simulink model "arduino_I2C_hmc5983"  (R2019b)
settings: Solver=FixedStepAuto  StartTime=0.0  StopTime=120  RelTol=1e-3  EnableMultiTasking=on
model workspace (MAT data in the model file):
  craVal = 144
  crbVal = 224
  modeVal = 0
  slaveaddress = 30
libraries: arduinolib x18, simulink x1
settings Model: SILPILModeSetting=veronly  ExtModeTrigDuration=2  OrderedModelArguments=off  Creator=Hirotoshi Maeda  LastModifiedBy=Hirotoshi Maeda
settings OptimizationCC: EnhancedBackFolding=on  PassReuseOutputArgsAs=Individual arguments  ZeroExternalMemoryAtStartup=off  ZeroInternalMemoryAtStartup=off  MaxStackSize=64  OptimizeBlockOrder=speed  DifferentSizesBufferReuse=on  OptimizationCustomize=off  EfficientTunableParamExpr=on
settings DebuggingCC: ParameterTunabilityLossMsg=error
settings HardwareCC: ProdBitPerInt=16  ProdBitPerPointer=16  ProdBitPerSizeT=16  ProdBitPerPtrDiffT=16  ProdLargestAtomicFloat=None  ProdWordSize=8  ProdHWDeviceType=Atmel->AVR  UseSimulinkCoderFeatures=off
settings SFSimCC: MATLABDynamicMemAlloc=off
settings RTWCC: SystemTargetFile=ert.tlc  HardwareBoard=Arduino Uno  TLCOptions=-aInlineSetEventsForThisBaseRateFcn=TLC_FALSE -aSuppressMultiTaskScheduler=TLC_FALSE -aRateBasedStepFcn=1  TemplateMakefile=ert_default_tmf  RTWVerbose=off  Toolchain=Arduino AVR  BuildConfiguration=Faster Runs  IncludeHyperlinkInReport=on
settings CodeAppCC: ForceParamTrailComments=on  OperatorAnnotations=on  SimulinkDataObjDesc=on  SFDataObjDesc=on  MangleLength=10  InsertBlockDesc=on
settings ERTTargetCC: SupportContinuousTime=on  SupportVariableSizeSignals=on  ExtMode=on  ExtModeStaticAllocSize=250  ExtModeMexArgs='127.0.0.1' 0 17725  ERTSrcFileBannerTemplate=codertarget_code_template.cgt  ERTHdrFileBannerTemplate=codertarget_code_template.cgt  ERTDataSrcFileTemplate=codertarget_code_template.cgt  ERTDataHdrFileTemplate=codertarget_code_template.cgt

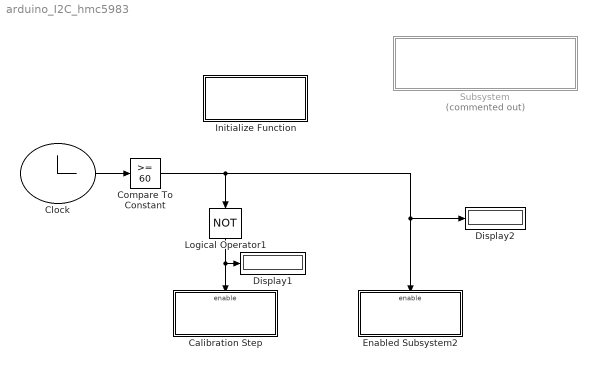
== system arduino_I2C_hmc5983 ==
  "Calibration Step " : Subsystem  Priority=3  TreatAsAtomicUnit=on
  Clock : Clock
  Compare To Constant : simulink/Logic and Bit Operations/Compare To Constant  relop=>=  const=60  OutDataTypeStr=boolean
  Display1 : Display
  Display2 : Display
  Enabled Subsystem2 : Subsystem  Priority=3  TreatAsAtomicUnit=on
  Initialize Function : Subsystem  TreatAsAtomicUnit=on
  Logical Operator1 : Logic  Operator=NOT  AllPortsSameDT=off  OutDataTypeStr=boolean
  Subsystem : Subsystem  Commented=on
  wires:
  Compare To Constant/1 -> Logical Operator1/1, Enabled Subsystem2/Enable, Display2/1
  Clock/1 -> Compare To Constant/1
  Logical Operator1/1 -> "Calibration Step "/Enable, Display1/1

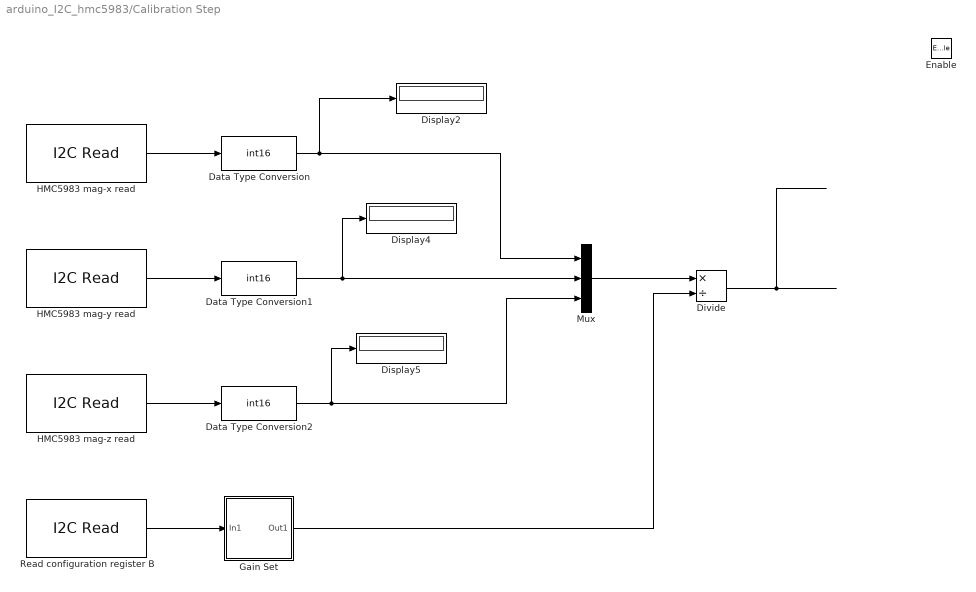
== system arduino_I2C_hmc5983/Calibration Step  ==
  Enable : EnablePort
  Data Type Conversion : DataTypeConversion  OutDataTypeStr=int16
  Data Type Conversion1 : DataTypeConversion  OutDataTypeStr=int16
  Data Type Conversion2 : DataTypeConversion  OutDataTypeStr=int16
  Display2 : Display
      settings: Format=hex (Stored Integer)
  Display4 : Display
      settings: Format=hex (Stored Integer)
  Display5 : Display
      settings: Format=hex (Stored Integer)
  Divide : Product  Inputs=*/
  Gain Set : Subsystem
  HMC5983 mag-x read : arduinolib/I2C Read  I2CModule=0  Mode=Master  SlaveAddress=slaveaddress  SlaveByteOrder=BigEndian  Direction=Receiver  RegisterAddressMode=on  RegisterAddress=hex2dec('03')  SlaveDataType=int16  DataLength=1  NoAck=off  RepeatedStart=off  OutputStatus=off  blockPlatform=ARDUINO  SampleTime=.1
      settings: SourceProductName=Simulink Support Package for Arduino Hardware  SourceProductBaseCode=ARDUINO
  HMC5983 mag-y read : arduinolib/I2C Read  I2CModule=0  Mode=Master  SlaveAddress=slaveaddress  SlaveByteOrder=BigEndian  Direction=Receiver  RegisterAddressMode=on  RegisterAddress=hex2dec('07')  SlaveDataType=int16  DataLength=1  NoAck=off  RepeatedStart=off  OutputStatus=off  blockPlatform=ARDUINO  SampleTime=.1
      settings: SourceProductName=Simulink Support Package for Arduino Hardware  SourceProductBaseCode=ARDUINO
  HMC5983 mag-z read : arduinolib/I2C Read  I2CModule=0  Mode=Master  SlaveAddress=slaveaddress  SlaveByteOrder=BigEndian  Direction=Receiver  RegisterAddressMode=on  RegisterAddress=hex2dec('05')  SlaveDataType=int16  DataLength=1  NoAck=off  RepeatedStart=off  OutputStatus=off  blockPlatform=ARDUINO  SampleTime=.1
      settings: SourceProductName=Simulink Support Package for Arduino Hardware  SourceProductBaseCode=ARDUINO
  Mux : Mux  Inputs=3
  Read configuration register B : arduinolib/I2C Read  I2CModule=0  Mode=Master  SlaveAddress=slaveaddress  SlaveByteOrder=BigEndian  Direction=Receiver  RegisterAddressMode=on  RegisterAddress=hex2dec('01')  SlaveDataType=uint8  DataLength=1  NoAck=off  RepeatedStart=off  OutputStatus=off  blockPlatform=ARDUINO  SampleTime=.1
      settings: SourceProductName=Simulink Support Package for Arduino Hardware  SourceProductBaseCode=ARDUINO
  wires:
  Mux/1 -> Divide/1
  Divide/1 -> ?
  HMC5983 mag-z read/1 -> Data Type Conversion2/1
  HMC5983 mag-y read/1 -> Data Type Conversion1/1
  HMC5983 mag-x read/1 -> Data Type Conversion/1
  Data Type Conversion/1 -> Mux/1, Display2/1
  Data Type Conversion1/1 -> Mux/2, Display4/1
  Data Type Conversion2/1 -> Display5/1, Mux/3
  Gain Set/1(Out1) -> Divide/2
  Read configuration register B/1 -> Gain Set/1(In1)

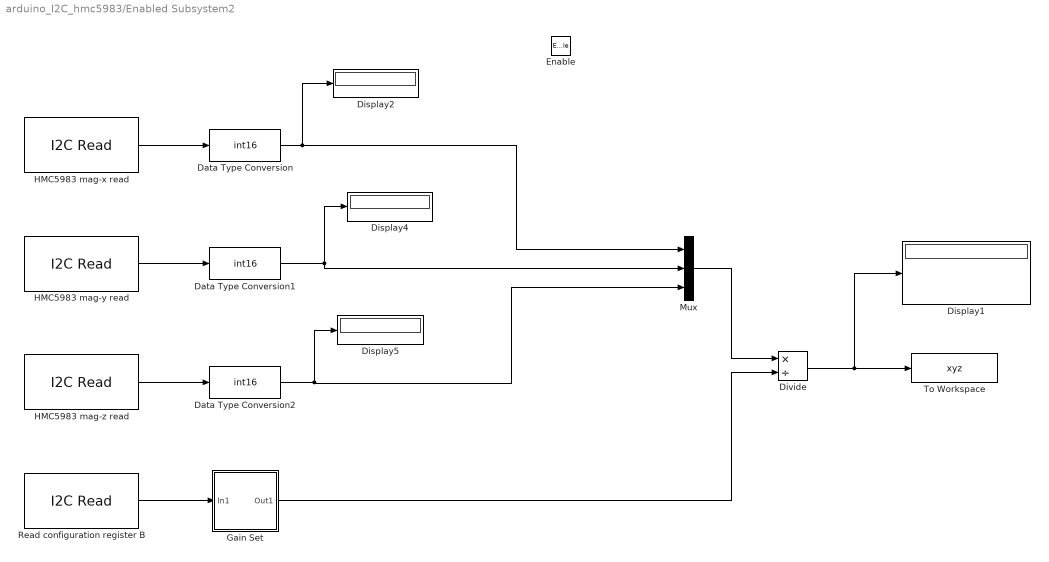
== system arduino_I2C_hmc5983/Enabled Subsystem2 ==
  Enable : EnablePort
  Data Type Conversion : DataTypeConversion  OutDataTypeStr=int16
  Data Type Conversion1 : DataTypeConversion  OutDataTypeStr=int16
  Data Type Conversion2 : DataTypeConversion  OutDataTypeStr=int16
  Display{1..2,4..5} (4 alike) : Display
      settings: Format=hex (Stored Integer)
  Divide : Product  Inputs=*/
  Gain Set : Subsystem
  HMC5983 mag-x read : arduinolib/I2C Read  I2CModule=0  Mode=Master  SlaveAddress=slaveaddress  SlaveByteOrder=BigEndian  Direction=Receiver  RegisterAddressMode=on  RegisterAddress=hex2dec('03')  SlaveDataType=int16  DataLength=1  NoAck=off  RepeatedStart=off  OutputStatus=off  blockPlatform=ARDUINO  SampleTime=.1
      settings: SourceProductName=Simulink Support Package for Arduino Hardware  SourceProductBaseCode=ARDUINO
  HMC5983 mag-y read : arduinolib/I2C Read  I2CModule=0  Mode=Master  SlaveAddress=slaveaddress  SlaveByteOrder=BigEndian  Direction=Receiver  RegisterAddressMode=on  RegisterAddress=hex2dec('07')  SlaveDataType=int16  DataLength=1  NoAck=off  RepeatedStart=off  OutputStatus=off  blockPlatform=ARDUINO  SampleTime=.1
      settings: SourceProductName=Simulink Support Package for Arduino Hardware  SourceProductBaseCode=ARDUINO
  HMC5983 mag-z read : arduinolib/I2C Read  I2CModule=0  Mode=Master  SlaveAddress=slaveaddress  SlaveByteOrder=BigEndian  Direction=Receiver  RegisterAddressMode=on  RegisterAddress=hex2dec('05')  SlaveDataType=int16  DataLength=1  NoAck=off  RepeatedStart=off  OutputStatus=off  blockPlatform=ARDUINO  SampleTime=.1
      settings: SourceProductName=Simulink Support Package for Arduino Hardware  SourceProductBaseCode=ARDUINO
  Mux : Mux  Inputs=3
  Read configuration register B : arduinolib/I2C Read  I2CModule=0  Mode=Master  SlaveAddress=slaveaddress  SlaveByteOrder=BigEndian  Direction=Receiver  RegisterAddressMode=on  RegisterAddress=hex2dec('01')  SlaveDataType=uint8  DataLength=1  NoAck=off  RepeatedStart=off  OutputStatus=off  blockPlatform=ARDUINO  SampleTime=.1
      settings: SourceProductName=Simulink Support Package for Arduino Hardware  SourceProductBaseCode=ARDUINO
  To Workspace : ToWorkspace  VariableName=xyz  SaveFormat=Timeseries  SampleTime=-1
  wires:
  Mux/1 -> Divide/1
  Divide/1 -> To Workspace/1, Display1/1
  HMC5983 mag-z read/1 -> Data Type Conversion2/1
  HMC5983 mag-y read/1 -> Data Type Conversion1/1
  HMC5983 mag-x read/1 -> Data Type Conversion/1
  Data Type Conversion/1 -> Mux/1, Display2/1
  Data Type Conversion1/1 -> Mux/2, Display4/1
  Data Type Conversion2/1 -> Display5/1, Mux/3
  Gain Set/1(Out1) -> Divide/2
  Read configuration register B/1 -> Gain Set/1(In1)

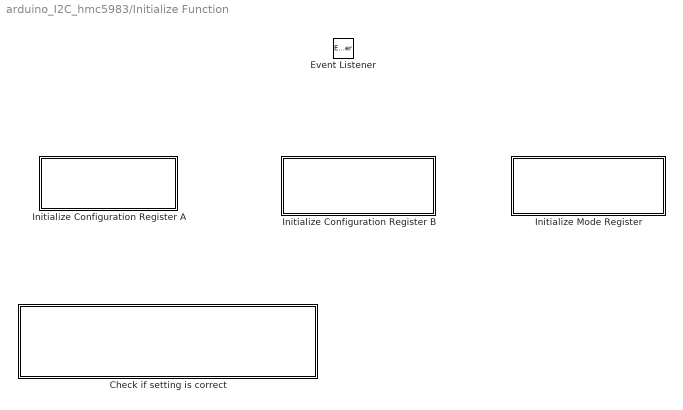
== system arduino_I2C_hmc5983/Initialize Function ==
  "Check if setting is correct " : Subsystem  Priority=2
  Event Listener : EventListener  DisableCoverage=on  EventName=reset
  Initialize Configuration Register A : Subsystem  Priority=1
  Initialize Configuration Register B : Subsystem  Priority=1
  "Initialize Mode Register " : Subsystem  Priority=1

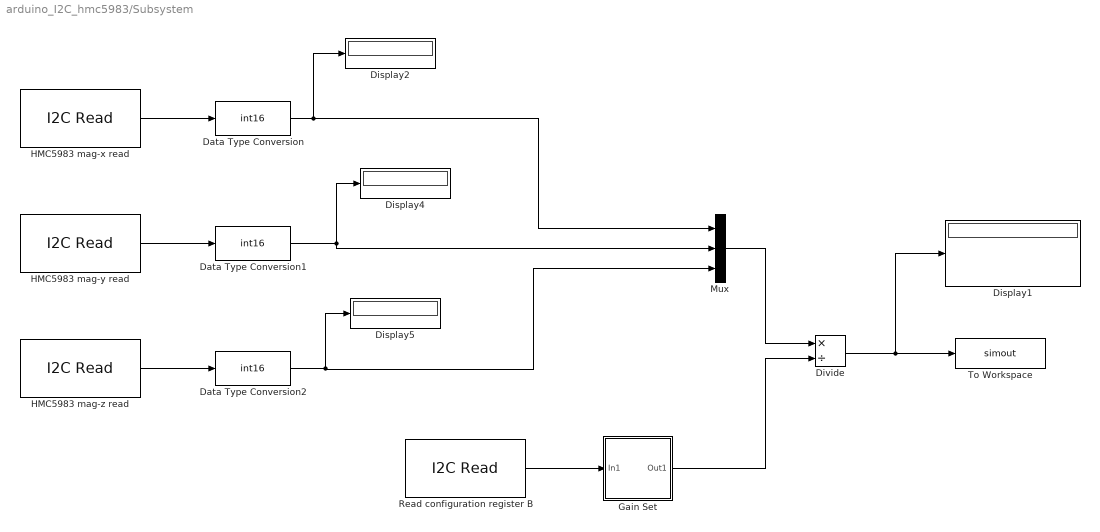
== system arduino_I2C_hmc5983/Subsystem ==
  Data Type Conversion : DataTypeConversion  OutDataTypeStr=int16
  Data Type Conversion1 : DataTypeConversion  OutDataTypeStr=int16
  Data Type Conversion2 : DataTypeConversion  OutDataTypeStr=int16
  Display{1..2,4..5} (4 alike) : Display
      settings: Format=hex (Stored Integer)
  Divide : Product  Inputs=*/
  Gain Set : Subsystem
  HMC5983 mag-x read : arduinolib/I2C Read  I2CModule=0  Mode=Master  SlaveAddress=slaveaddress  SlaveByteOrder=BigEndian  Direction=Receiver  RegisterAddressMode=on  RegisterAddress=hex2dec('03')  SlaveDataType=int16  DataLength=1  NoAck=off  RepeatedStart=off  OutputStatus=off  blockPlatform=ARDUINO  SampleTime=.1
      settings: SourceProductName=Simulink Support Package for Arduino Hardware  SourceProductBaseCode=ARDUINO
  HMC5983 mag-y read : arduinolib/I2C Read  I2CModule=0  Mode=Master  SlaveAddress=slaveaddress  SlaveByteOrder=BigEndian  Direction=Receiver  RegisterAddressMode=on  RegisterAddress=hex2dec('07')  SlaveDataType=int16  DataLength=1  NoAck=off  RepeatedStart=off  OutputStatus=off  blockPlatform=ARDUINO  SampleTime=.1
      settings: SourceProductName=Simulink Support Package for Arduino Hardware  SourceProductBaseCode=ARDUINO
  HMC5983 mag-z read : arduinolib/I2C Read  I2CModule=0  Mode=Master  SlaveAddress=slaveaddress  SlaveByteOrder=BigEndian  Direction=Receiver  RegisterAddressMode=on  RegisterAddress=hex2dec('05')  SlaveDataType=int16  DataLength=1  NoAck=off  RepeatedStart=off  OutputStatus=off  blockPlatform=ARDUINO  SampleTime=.1
      settings: SourceProductName=Simulink Support Package for Arduino Hardware  SourceProductBaseCode=ARDUINO
  Mux : Mux  Inputs=3
  Read configuration register B : arduinolib/I2C Read  I2CModule=0  Mode=Master  SlaveAddress=slaveaddress  SlaveByteOrder=BigEndian  Direction=Receiver  RegisterAddressMode=on  RegisterAddress=hex2dec('01')  SlaveDataType=uint8  DataLength=1  NoAck=off  RepeatedStart=off  OutputStatus=off  blockPlatform=ARDUINO  SampleTime=inf
      settings: SourceProductName=Simulink Support Package for Arduino Hardware  SourceProductBaseCode=ARDUINO
  To Workspace : ToWorkspace  VariableName=simout  SaveFormat=Timeseries  SampleTime=-1
  wires:
  Data Type Conversion2/1 -> Display5/1, Mux/3
  Data Type Conversion1/1 -> Mux/2, Display4/1
  HMC5983 mag-x read/1 -> Data Type Conversion/1
  HMC5983 mag-z read/1 -> Data Type Conversion2/1
  Data Type Conversion/1 -> Mux/1, Display2/1
  HMC5983 mag-y read/1 -> Data Type Conversion1/1
  Mux/1 -> Divide/1
  Read configuration register B/1 -> Gain Set/1(In1)
  Gain Set/1(Out1) -> Divide/2
  Divide/1 -> To Workspace/1, Display1/1

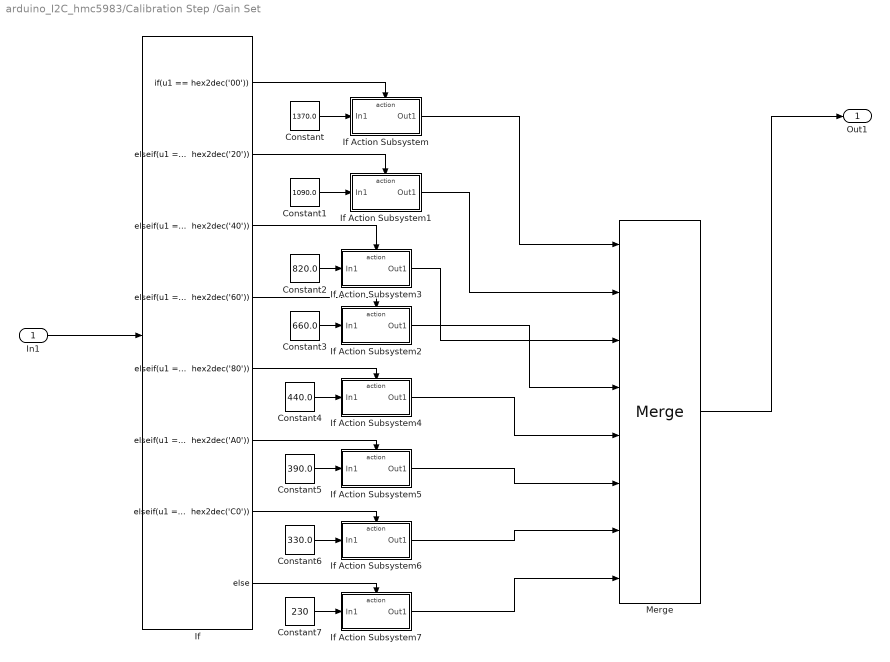
== system arduino_I2C_hmc5983/Calibration Step /Gain Set ==
  In1 : Inport
  Constant : Constant  Value=1370.0
  Constant1 : Constant  Value=1090.0
  Constant2 : Constant  Value=820.0
  Constant3 : Constant  Value=660.0
  Constant4 : Constant  Value=440.0
  Constant5 : Constant  Value=390.0
  Constant6 : Constant  Value=330.0
  Constant7 : Constant  Value=230
  If : If  IfExpression=u1 == hex2dec('00')  ElseIfExpressions="u1 ==  hex2dec('20'), u1 ==  hex2dec('40'), u1 ==  hex2dec('60'), u1 ==  hex2dec('80'), u1 ==  hex2dec('A0'), u1 ==  hex2dec('C0')"
  If Action Subsystem : Subsystem  TreatAsAtomicUnit=on
  If Action Subsystem1 : Subsystem  TreatAsAtomicUnit=on
  If Action Subsystem2 : Subsystem  TreatAsAtomicUnit=on
  If Action Subsystem3 : Subsystem  TreatAsAtomicUnit=on
  If Action Subsystem4 : Subsystem  TreatAsAtomicUnit=on
  If Action Subsystem5 : Subsystem  TreatAsAtomicUnit=on
  If Action Subsystem6 : Subsystem  TreatAsAtomicUnit=on
  If Action Subsystem7 : Subsystem  TreatAsAtomicUnit=on
  Merge : Merge  Inputs=8
  Out1 : Outport
  wires:
  Constant7/1 -> If Action Subsystem7/1(In1)
  If/6 -> If Action Subsystem5/Action
  Constant6/1 -> If Action Subsystem6/1(In1)
  If Action Subsystem/1(Out1) -> Merge/1
  Constant1/1 -> If Action Subsystem1/1(In1)
  If/3 -> If Action Subsystem3/Action
  If/4 -> If Action Subsystem2/Action
  If Action Subsystem6/1(Out1) -> Merge/7
  Constant4/1 -> If Action Subsystem4/1(In1)
  If/2 -> If Action Subsystem1/Action
  If/5 -> If Action Subsystem4/Action
  Merge/1 -> Out1/1
  Constant/1 -> If Action Subsystem/1(In1)
  If Action Subsystem1/1(Out1) -> Merge/2
  If/8 -> If Action Subsystem7/Action
  Constant2/1 -> If Action Subsystem3/1(In1)
  Constant3/1 -> If Action Subsystem2/1(In1)
  If Action Subsystem7/1(Out1) -> Merge/8
  If Action Subsystem2/1(Out1) -> Merge/4
  If Action Subsystem4/1(Out1) -> Merge/5
  If Action Subsystem5/1(Out1) -> Merge/6
  If/7 -> If Action Subsystem6/Action
  If Action Subsystem3/1(Out1) -> Merge/3
  If/1 -> If Action Subsystem/Action
  Constant5/1 -> If Action Subsystem5/1(In1)
  In1/1 -> If/1

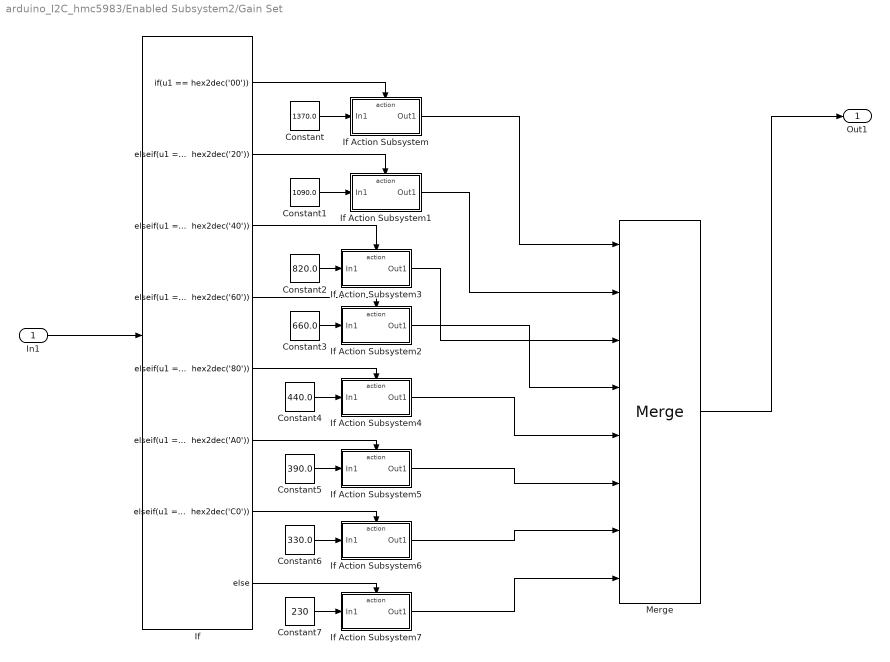
== system arduino_I2C_hmc5983/Enabled Subsystem2/Gain Set ==
  In1 : Inport
  Constant : Constant  Value=1370.0
  Constant1 : Constant  Value=1090.0
  Constant2 : Constant  Value=820.0
  Constant3 : Constant  Value=660.0
  Constant4 : Constant  Value=440.0
  Constant5 : Constant  Value=390.0
  Constant6 : Constant  Value=330.0
  Constant7 : Constant  Value=230
  If : If  IfExpression=u1 == hex2dec('00')  ElseIfExpressions="u1 ==  hex2dec('20'), u1 ==  hex2dec('40'), u1 ==  hex2dec('60'), u1 ==  hex2dec('80'), u1 ==  hex2dec('A0'), u1 ==  hex2dec('C0')"
  If Action Subsystem : Subsystem  TreatAsAtomicUnit=on
  If Action Subsystem1 : Subsystem  TreatAsAtomicUnit=on
  If Action Subsystem2 : Subsystem  TreatAsAtomicUnit=on
  If Action Subsystem3 : Subsystem  TreatAsAtomicUnit=on
  If Action Subsystem4 : Subsystem  TreatAsAtomicUnit=on
  If Action Subsystem5 : Subsystem  TreatAsAtomicUnit=on
  If Action Subsystem6 : Subsystem  TreatAsAtomicUnit=on
  If Action Subsystem7 : Subsystem  TreatAsAtomicUnit=on
  Merge : Merge  Inputs=8
  Out1 : Outport
  wires:
  Constant7/1 -> If Action Subsystem7/1(In1)
  If/6 -> If Action Subsystem5/Action
  Constant6/1 -> If Action Subsystem6/1(In1)
  If Action Subsystem/1(Out1) -> Merge/1
  Constant1/1 -> If Action Subsystem1/1(In1)
  If/3 -> If Action Subsystem3/Action
  If/4 -> If Action Subsystem2/Action
  If Action Subsystem6/1(Out1) -> Merge/7
  Constant4/1 -> If Action Subsystem4/1(In1)
  If/2 -> If Action Subsystem1/Action
  If/5 -> If Action Subsystem4/Action
  Merge/1 -> Out1/1
  Constant/1 -> If Action Subsystem/1(In1)
  If Action Subsystem1/1(Out1) -> Merge/2
  If/8 -> If Action Subsystem7/Action
  Constant2/1 -> If Action Subsystem3/1(In1)
  Constant3/1 -> If Action Subsystem2/1(In1)
  If Action Subsystem7/1(Out1) -> Merge/8
  If Action Subsystem2/1(Out1) -> Merge/4
  If Action Subsystem4/1(Out1) -> Merge/5
  If Action Subsystem5/1(Out1) -> Merge/6
  If/7 -> If Action Subsystem6/Action
  If Action Subsystem3/1(Out1) -> Merge/3
  If/1 -> If Action Subsystem/Action
  Constant5/1 -> If Action Subsystem5/1(In1)
  In1/1 -> If/1

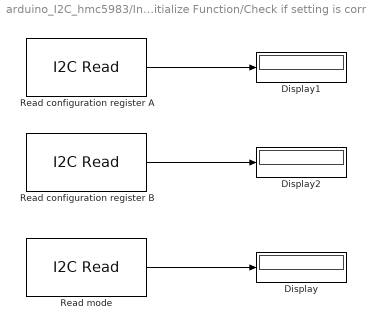
== system arduino_I2C_hmc5983/Initialize Function/Check if setting is correct  ==
  Display : Display
      settings: Format=hex (Stored Integer)
  Display1 : Display
      settings: Format=hex (Stored Integer)
  Display2 : Display
      settings: Format=hex (Stored Integer)
  Read configuration register A : arduinolib/I2C Read  Priority=2  I2CModule=0  Mode=Master  SlaveAddress=slaveaddress  SlaveByteOrder=BigEndian  Direction=Receiver  RegisterAddressMode=on  RegisterAddress=hex2dec('00')  SlaveDataType=int8  DataLength=1  NoAck=off  RepeatedStart=off  OutputStatus=off  blockPlatform=ARDUINO  SampleTime=inf
      settings: SourceProductName=Simulink Support Package for Arduino Hardware  SourceProductBaseCode=ARDUINO
  Read configuration register B : arduinolib/I2C Read  Priority=2  I2CModule=0  Mode=Master  SlaveAddress=slaveaddress  SlaveByteOrder=BigEndian  Direction=Receiver  RegisterAddressMode=on  RegisterAddress=hex2dec('01')  SlaveDataType=int8  DataLength=1  NoAck=off  RepeatedStart=off  OutputStatus=off  blockPlatform=ARDUINO  SampleTime=inf
      settings: SourceProductName=Simulink Support Package for Arduino Hardware  SourceProductBaseCode=ARDUINO
  "Read mode " : arduinolib/I2C Read  Priority=2  I2CModule=0  Mode=Master  SlaveAddress=slaveaddress  SlaveByteOrder=BigEndian  Direction=Receiver  RegisterAddressMode=on  RegisterAddress=hex2dec('02')  SlaveDataType=int8  DataLength=1  NoAck=off  RepeatedStart=off  OutputStatus=off  blockPlatform=ARDUINO  SampleTime=inf
      settings: SourceProductName=Simulink Support Package for Arduino Hardware  SourceProductBaseCode=ARDUINO
  wires:
  "Read mode "/1 -> Display/1
  Read configuration register B/1 -> Display2/1
  Read configuration register A/1 -> Display1/1

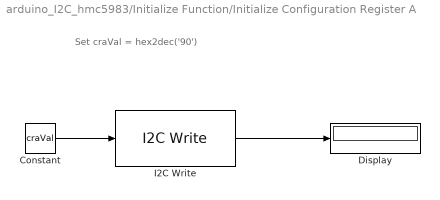
== system arduino_I2C_hmc5983/Initialize Function/Initialize Configuration Register A ==
  note: Set craVal = hex2dec('90')
  Constant : Constant  Value=craVal  OutDataTypeStr=uint8
  Display : Display
  I2C Write : arduinolib/I2C Write  I2CModule=0  Mode=Master  SlaveAddress=slaveaddress  SlaveByteOrder=BigEndian  Direction=Transmitter  RegisterAddressMode=on  RegisterAddress=hex2dec('00')  SlaveDataType=uint8  DataLength=1  NoAck=off  RepeatedStart=off  OutputStatus=on  blockPlatform=ARDUINO
      settings: SourceProductName=Simulink Support Package for Arduino Hardware  SourceProductBaseCode=ARDUINO
  wires:
  Constant/1 -> I2C Write/1
  I2C Write/1 -> Display/1

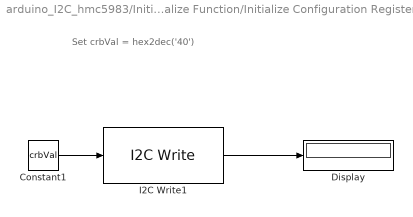
== system arduino_I2C_hmc5983/Initialize Function/Initialize Configuration Register B ==
  note: Set crbVal = hex2dec('40')
  Constant1 : Constant  Value=crbVal  OutDataTypeStr=uint8
  Display : Display
  I2C Write1 : arduinolib/I2C Write  I2CModule=0  Mode=Master  SlaveAddress=slaveaddress  SlaveByteOrder=BigEndian  Direction=Transmitter  RegisterAddressMode=on  RegisterAddress=hex2dec('01')  SlaveDataType=uint8  DataLength=1  NoAck=off  RepeatedStart=off  OutputStatus=on  blockPlatform=ARDUINO
      settings: SourceProductName=Simulink Support Package for Arduino Hardware  SourceProductBaseCode=ARDUINO
  wires:
  Constant1/1 -> I2C Write1/1
  I2C Write1/1 -> Display/1

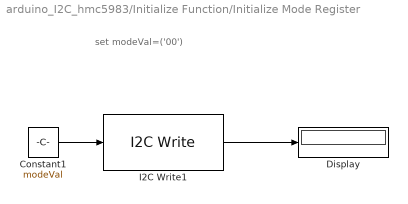
== system arduino_I2C_hmc5983/Initialize Function/Initialize Mode Register  ==
  note: set modeVal=('00')
  Constant1 : Constant  Value=modeVal  OutDataTypeStr=uint8
  Display : Display
  I2C Write1 : arduinolib/I2C Write  I2CModule=0  Mode=Master  SlaveAddress=slaveaddress  SlaveByteOrder=BigEndian  Direction=Transmitter  RegisterAddressMode=on  RegisterAddress=hex2dec('02')  SlaveDataType=uint8  DataLength=1  NoAck=off  RepeatedStart=off  OutputStatus=on  blockPlatform=ARDUINO
      settings: SourceProductName=Simulink Support Package for Arduino Hardware  SourceProductBaseCode=ARDUINO
  wires:
  Constant1/1 -> I2C Write1/1
  I2C Write1/1 -> Display/1

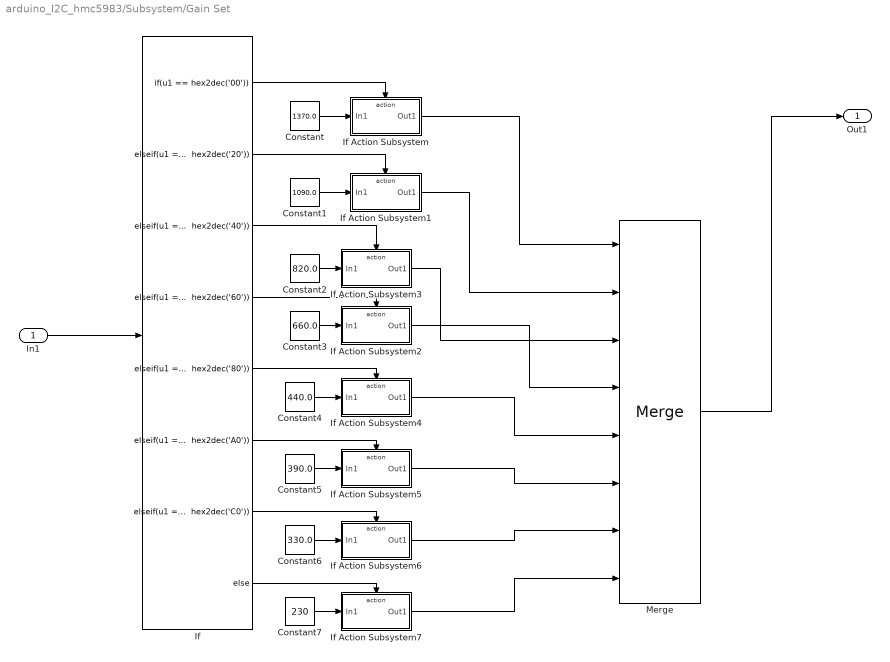
== system arduino_I2C_hmc5983/Subsystem/Gain Set ==
  In1 : Inport
  Constant : Constant  Value=1370.0
  Constant1 : Constant  Value=1090.0
  Constant2 : Constant  Value=820.0
  Constant3 : Constant  Value=660.0
  Constant4 : Constant  Value=440.0
  Constant5 : Constant  Value=390.0
  Constant6 : Constant  Value=330.0
  Constant7 : Constant  Value=230
  If : If  IfExpression=u1 == hex2dec('00')  ElseIfExpressions="u1 ==  hex2dec('20'), u1 ==  hex2dec('40'), u1 ==  hex2dec('60'), u1 ==  hex2dec('80'), u1 ==  hex2dec('A0'), u1 ==  hex2dec('C0')"
  If Action Subsystem : Subsystem  TreatAsAtomicUnit=on
  If Action Subsystem1 : Subsystem  TreatAsAtomicUnit=on
  If Action Subsystem2 : Subsystem  TreatAsAtomicUnit=on
  If Action Subsystem3 : Subsystem  TreatAsAtomicUnit=on
  If Action Subsystem4 : Subsystem  TreatAsAtomicUnit=on
  If Action Subsystem5 : Subsystem  TreatAsAtomicUnit=on
  If Action Subsystem6 : Subsystem  TreatAsAtomicUnit=on
  If Action Subsystem7 : Subsystem  TreatAsAtomicUnit=on
  Merge : Merge  Inputs=8
  Out1 : Outport
  wires:
  Constant7/1 -> If Action Subsystem7/1(In1)
  If/6 -> If Action Subsystem5/Action
  Constant6/1 -> If Action Subsystem6/1(In1)
  If Action Subsystem/1(Out1) -> Merge/1
  Constant1/1 -> If Action Subsystem1/1(In1)
  If/3 -> If Action Subsystem3/Action
  If/4 -> If Action Subsystem2/Action
  If Action Subsystem6/1(Out1) -> Merge/7
  Constant4/1 -> If Action Subsystem4/1(In1)
  If/2 -> If Action Subsystem1/Action
  If/5 -> If Action Subsystem4/Action
  Merge/1 -> Out1/1
  Constant/1 -> If Action Subsystem/1(In1)
  If Action Subsystem1/1(Out1) -> Merge/2
  If/8 -> If Action Subsystem7/Action
  Constant2/1 -> If Action Subsystem3/1(In1)
  Constant3/1 -> If Action Subsystem2/1(In1)
  If Action Subsystem7/1(Out1) -> Merge/8
  If Action Subsystem2/1(Out1) -> Merge/4
  If Action Subsystem4/1(Out1) -> Merge/5
  If Action Subsystem5/1(Out1) -> Merge/6
  If/7 -> If Action Subsystem6/Action
  If Action Subsystem3/1(Out1) -> Merge/3
  If/1 -> If Action Subsystem/Action
  Constant5/1 -> If Action Subsystem5/1(In1)
  In1/1 -> If/1

== system arduino_I2C_hmc5983/Calibration Step /Gain Set/If Action Subsystem ==
  In1 : Inport
  Action Port : ActionPort  ActionPortLabel=if(u1 == hex2dec('00'))
  Out1 : Outport
  wires:
  In1/1 -> Out1/1

== system arduino_I2C_hmc5983/Calibration Step /Gain Set/If Action Subsystem1 ==
  In1 : Inport
  Action Port : ActionPort  ActionPortLabel="elseif(u1 ==  hex2dec('20'))"
  Out1 : Outport
  wires:
  In1/1 -> Out1/1

== system arduino_I2C_hmc5983/Calibration Step /Gain Set/If Action Subsystem2 ==
  In1 : Inport
  Action Port : ActionPort  ActionPortLabel="elseif( u1 ==  hex2dec('60'))"
  Out1 : Outport
  wires:
  In1/1 -> Out1/1

== system arduino_I2C_hmc5983/Calibration Step /Gain Set/If Action Subsystem3 ==
  In1 : Inport
  Action Port : ActionPort  ActionPortLabel="elseif( u1 ==  hex2dec('40'))"
  Out1 : Outport
  wires:
  In1/1 -> Out1/1

== system arduino_I2C_hmc5983/Calibration Step /Gain Set/If Action Subsystem4 ==
  In1 : Inport
  Action Port : ActionPort  ActionPortLabel="elseif( u1 ==  hex2dec('80'))"
  Out1 : Outport
  wires:
  In1/1 -> Out1/1

== system arduino_I2C_hmc5983/Calibration Step /Gain Set/If Action Subsystem5 ==
  In1 : Inport
  Action Port : ActionPort  ActionPortLabel="elseif( u1 ==  hex2dec('A0'))"
  Out1 : Outport
  wires:
  In1/1 -> Out1/1

== system arduino_I2C_hmc5983/Calibration Step /Gain Set/If Action Subsystem6 ==
  In1 : Inport
  Action Port : ActionPort  ActionPortLabel="elseif( u1 ==  hex2dec('C0'))"
  Out1 : Outport
  wires:
  In1/1 -> Out1/1

== system arduino_I2C_hmc5983/Calibration Step /Gain Set/If Action Subsystem7 ==
  In1 : Inport
  Action Port : ActionPort  ActionPortLabel=else
  Out1 : Outport
  wires:
  In1/1 -> Out1/1

== system arduino_I2C_hmc5983/Enabled Subsystem2/Gain Set/If Action Subsystem ==
  In1 : Inport
  Action Port : ActionPort  ActionPortLabel=if(u1 == hex2dec('00'))
  Out1 : Outport
  wires:
  In1/1 -> Out1/1

== system arduino_I2C_hmc5983/Enabled Subsystem2/Gain Set/If Action Subsystem1 ==
  In1 : Inport
  Action Port : ActionPort  ActionPortLabel="elseif(u1 ==  hex2dec('20'))"
  Out1 : Outport
  wires:
  In1/1 -> Out1/1

== system arduino_I2C_hmc5983/Enabled Subsystem2/Gain Set/If Action Subsystem2 ==
  In1 : Inport
  Action Port : ActionPort  ActionPortLabel="elseif( u1 ==  hex2dec('60'))"
  Out1 : Outport
  wires:
  In1/1 -> Out1/1

== system arduino_I2C_hmc5983/Enabled Subsystem2/Gain Set/If Action Subsystem3 ==
  In1 : Inport
  Action Port : ActionPort  ActionPortLabel="elseif( u1 ==  hex2dec('40'))"
  Out1 : Outport
  wires:
  In1/1 -> Out1/1

== system arduino_I2C_hmc5983/Enabled Subsystem2/Gain Set/If Action Subsystem4 ==
  In1 : Inport
  Action Port : ActionPort  ActionPortLabel="elseif( u1 ==  hex2dec('80'))"
  Out1 : Outport
  wires:
  In1/1 -> Out1/1

== system arduino_I2C_hmc5983/Enabled Subsystem2/Gain Set/If Action Subsystem5 ==
  In1 : Inport
  Action Port : ActionPort  ActionPortLabel="elseif( u1 ==  hex2dec('A0'))"
  Out1 : Outport
  wires:
  In1/1 -> Out1/1

== system arduino_I2C_hmc5983/Enabled Subsystem2/Gain Set/If Action Subsystem6 ==
  In1 : Inport
  Action Port : ActionPort  ActionPortLabel="elseif( u1 ==  hex2dec('C0'))"
  Out1 : Outport
  wires:
  In1/1 -> Out1/1

== system arduino_I2C_hmc5983/Enabled Subsystem2/Gain Set/If Action Subsystem7 ==
  In1 : Inport
  Action Port : ActionPort  ActionPortLabel=else
  Out1 : Outport
  wires:
  In1/1 -> Out1/1

== system arduino_I2C_hmc5983/Subsystem/Gain Set/If Action Subsystem ==
  In1 : Inport
  Action Port : ActionPort  ActionPortLabel=if(u1 == hex2dec('00'))
  Out1 : Outport
  wires:
  In1/1 -> Out1/1

== system arduino_I2C_hmc5983/Subsystem/Gain Set/If Action Subsystem1 ==
  In1 : Inport
  Action Port : ActionPort  ActionPortLabel="elseif(u1 ==  hex2dec('20'))"
  Out1 : Outport
  wires:
  In1/1 -> Out1/1

== system arduino_I2C_hmc5983/Subsystem/Gain Set/If Action Subsystem2 ==
  In1 : Inport
  Action Port : ActionPort  ActionPortLabel="elseif( u1 ==  hex2dec('60'))"
  Out1 : Outport
  wires:
  In1/1 -> Out1/1

== system arduino_I2C_hmc5983/Subsystem/Gain Set/If Action Subsystem3 ==
  In1 : Inport
  Action Port : ActionPort  ActionPortLabel="elseif( u1 ==  hex2dec('40'))"
  Out1 : Outport
  wires:
  In1/1 -> Out1/1

== system arduino_I2C_hmc5983/Subsystem/Gain Set/If Action Subsystem4 ==
  In1 : Inport
  Action Port : ActionPort  ActionPortLabel="elseif( u1 ==  hex2dec('80'))"
  Out1 : Outport
  wires:
  In1/1 -> Out1/1

== system arduino_I2C_hmc5983/Subsystem/Gain Set/If Action Subsystem5 ==
  In1 : Inport
  Action Port : ActionPort  ActionPortLabel="elseif( u1 ==  hex2dec('A0'))"
  Out1 : Outport
  wires:
  In1/1 -> Out1/1

== system arduino_I2C_hmc5983/Subsystem/Gain Set/If Action Subsystem6 ==
  In1 : Inport
  Action Port : ActionPort  ActionPortLabel="elseif( u1 ==  hex2dec('C0'))"
  Out1 : Outport
  wires:
  In1/1 -> Out1/1

== system arduino_I2C_hmc5983/Subsystem/Gain Set/If Action Subsystem7 ==
  In1 : Inport
  Action Port : ActionPort  ActionPortLabel=else
  Out1 : Outport
  wires:
  In1/1 -> Out1/1
